simulink model "specificTaskTemplate"  (R2012b)
settings: Solver=FixedStepDiscrete  StartTime=0.0  StopTime=10.0  FixedStep=0.001  RelTol=1e-3
undefined symbols (not defined in the file): acquireMethods, clickPercentage, clickRefractoryPeriod, cuedText, cuedTextLength, cumulativeDwell, cursorDiameter, cursorDownColor, cursorNeuralColor, cursorNonneuralColor, displayShape, displayShape_1, displayShape_10, displayShape_2, displayShape_3, displayShape_4, displayShape_5, displayShape_6, displayShape_7, displayShape_8, displayShape_9, dwellRefractoryPeriod, gain, gloveBias, gloveLPDenominator, gloveLPNumerator, height, height_1, height_10, height_2, height_3, height_4, height_5, height_6, height_7, height_8, height_9, holdTime, ID, ID_1, ID_10, ID_2, ID_3, ID_4, ID_5, ID_6, ID_7, ID_8, ID_9, initialInput, initialLockout, initialState, inputType, keyboard, keyboardDims, keyPressedTime, maxTaskTime, mouseLPDenominator, mouseLPNumerator, mouseOffset ... (+122)
(part 2 of 2)

== matlab function specificTaskTemplate/keyboardTask ==
  data: xk input double size=[5 1]; behaviorPacket input Bus: behaviorPacketBus size=1; vizData input Bus: peripheralData; clickState input; clickParameters input; taskOutput output Bus: taskOutput; stateParameters input Bus: stateParams size=1; taskParameters input Bus: taskParamsBus; clock input; xpcTET input; keys input
function taskOutput  = keyboardTask(xk, behaviorPacket, vizData, clickState, clickParameters, stateParameters, taskParameters, clock, xpcTET, keys)
%#codegen

mouse = behaviorPacket.mouse(1:6);
glove = behaviorPacket.glove(1:5);
behaviorRequestClock = behaviorPacket.xpcRequestClock;
peripheralTimestamp = behaviorPacket.peripheralTimestamp(1:16);

%% CONSTANTS
TASK_NAME = 'keyboard';
VERSION_ID = single(2.010);
NUM_DIMS = double(DecoderConstants.NUM_KINEMATIC_DIMENSIONS);
STATEVEC_SIZE = 2*NUM_DIMS+1;
INIT_LENGTH = uint16(100); %ms
PRE_TRIAL_LENGTH = uint16(20); %ms
SCORE_LENGTH = uint16(4000); %ms
INIT_TIME = uint32(100);


%% INITIALIZE CURSOR TASK OUTPUT
fileLoggerData.data = uint8(zeros(1,1400));
fileLoggerData.dataLen = uint16(0);
fileLoggerData.fileName = uint8(zeros(1,20));
fileLoggerData.send = false;

fileLoggerFormat.format = uint8(zeros(1,1400));
fileLoggerFormat.formatLen = uint16(0);
fileLoggerFormat.fileName = uint8(zeros(1,20));

fileLoggerFormatAndData.format = fileLoggerFormat;
fileLoggerFormatAndData.data = fileLoggerData;

allowStop = true;
resetHMM = false;
taskOutput.flushFiles = false;
taskOutput.sendFormat = false;
taskOutput.taskDetails = fileLoggerFormat;
taskOutput.discrete = fileLoggerFormatAndData;
taskOutput.continuous = fileLoggerFormatAndData;
taskOutput.screen = fileLoggerFormatAndData;
taskOutput.sound = fileLoggerFormatAndData;
taskOutput.asynch = fileLoggerFormatAndData;
taskOutput.ttl = double(0);
taskOutput.xk = xk;
taskOutput.inputType = taskParameters.initialInput;
taskOutput.currentTarget = single(zeros([2 1]));
taskOutput.state = uint16(0);
taskOutput.paused = false;
taskOutput.allowStop = allowStop;
taskOutput.resetHMM = resetHMM;

%% TASK DETAILS PACKET
taskOutput.taskDetails = packFileLoggerTaskDetails(TASK_NAME, VERSION_ID, ...
    'STATE_INIT', uint8(KeyboardStates.STATE_INIT), ...
    'STATE_MOVE', uint8(KeyboardStates.STATE_MOVE),...
    'STATE_OVER_TARGET', uint8(KeyboardStates.STATE_OVER_TARGET),...
    'STATE_CLICK', uint8(KeyboardStates.STATE_CLICK),...
    'STATE_CLICK_REFRACTORY', uint8(KeyboardStates.STATE_CLICK_REFRACTORY),...
    'STATE_END', uint8(KeyboardStates.STATE_END),...
    'STATE_SHOW_SCORE', uint8(KeyboardStates.STATE_SHOW_SCORE),...
    'CLICK_IDLE', uint8(DiscreteStates.CLICK_IDLE),...
    'CLICK_MAIN', uint8(DiscreteStates.CLICK_MAIN),...
    'TASK_CUED_TEXT', uint8(keyboardConstants.TASK_CUED_TEXT), ...
    'TASK_FREE_TYPE', uint8(keyboardConstants.TASK_FREE_TYPE), ...
    'KEY_TYPE_LETTER', uint8(keyboardConstants.KEY_TYPE_LETTER), ...
    'KEY_TYPE_BACKSPACE', uint8(keyboardConstants.KEY_TYPE_BACKSPACE), ...
    'KEY_TYPE_SPACE', uint8(keyboardConstants.KEY_TYPE_SPACE), ...
    'KEY_TYPE_RETURN', uint8(keyboardConstants.KEY_TYPE_RETURN), ...
    'INPUT_TYPE_MOUSE_ABSOLUTE', uint8(cursorConstants.INPUT_TYPE_MOUSE_ABSOLUTE), ...
    'INPUT_TYPE_DECODE_V', uint8(cursorConstants.INPUT_TYPE_DECODE_V),...
    'CLICK_TYPE_NONE', uint8(clickConstants.CLICK_TYPE_NONE),...
    'CLICK_TYPE_GLOVE', uint8(clickConstants.CLICK_TYPE_GLOVE),...
    'CLICK_TYPE_NEURAL', uint8(clickConstants.CLICK_TYPE_NEURAL)...
);



%% DEFINE PERSISTENTS
persistent state vizPacket;
persistent pauseTriggered;
persistent stateTimer;
persistent holdTimer;
persistent cursorColor;

persistent trialNum;
persistent textInd;

persistent lockedParameters inputType;

persistent textSequence;
persistent previousOverTarget;
persistent selectedTarget;

persistent lastSoundTime lastSoundState lastAcquireMethod;

persistent totalTaskTime;

persistent lastResetTime lastResetState;
persistent initialClickTimer;

persistent lastEnteredCharacter;

%% store the amount of time dwelled on any target
persistent cumulativeDwell;

persistent lastRecenterTime lastRecenterSpot;

%% INITIALIZE PERSISTENTS
if(isempty(state))
    state = uint16(KeyboardStates.STATE_INIT);
    
    vizPacket = initVizPacket;
    stateTimer = uint16(0);
    holdTimer = uint16(0);
    pauseTriggered = true;
    
    cursorColor = double(zeros([3 1]));
    
    xk = double(zeros([STATEVEC_SIZE 1]));
    xk(end,1) = 1;
    
    %% buffer all the parameters off the bus
    lockedParameters = taskParameters;
    inputType = lockedParameters.initialInput;
    
    trialNum = uint16(1);
    textInd = uint16(1);
    previousOverTarget = uint16(0);
    selectedTarget = uint16(0);
    
    textSequence = zeros([1 uint16(keyboardConstants.MAX_CUED_TEXT)],'uint8');

    lastSoundTime = clock;
    lastSoundState = uint8(KeyboardStates.SOUND_STATE_IDLE);
    lastAcquireMethod = uint8(0);
    
    totalTaskTime = uint32(0);
    lastResetState = false;
    lastResetTime = uint32(0);
    initialClickTimer = uint16(0);
    lastEnteredCharacter = uint8(0);
    
	cumulativeDwell = initCumulativeDwell();
    lastRecenterTime = clock;
    lastRecenterSpot = [0;0];
end

%% trigger display resets on the rising edge of the parameter setting
resetDisplay = lockedParameters.resetDisplay;
if resetDisplay && ~lastResetState
    lastResetTime = clock;
end
lastResetState = resetDisplay;

if(clock < INIT_TIME)
    pauseTriggered = true;
end

if ~pauseTriggered
    totalTaskTime = totalTaskTime+1;
end
% We usually shouldn't write discrete data
writeDiscreteData = false;
writeContinuousData = true;

if(vizData.receive && (vizData.dataLen > 0 ))
    vizPacket = parseVizPacket(vizData.data);
end

isNeural = (uint16(inputType) == uint16(cursorConstants.INPUT_TYPE_DECODE_V));
isClicked = (uint16(clickState) == uint16(DiscreteStates.CLICK_MAIN));
isNone = (uint16(inputType) == uint16(cursorConstants.INPUT_TYPE_NONE));

%% set the cursor color 
%if isClicked
%    cursorColor(1:end) = taskParameters.cursorDownColor;
%else
if isNeural
    cursorColor(1:end) = taskParameters.cursorNeuralColor;
elseif isNone
    cursorColor(1:end) = [0; 204; 102;];
else
    cursorColor(1:end) = taskParameters.cursorNonneuralColor;
end

overTarget = uint16(0);
cuedTarget = uint16(0);
overCuedTarget = uint16(0);
cuedSuccess = uint8(0);
xkshift = xk(1:2)+[lockedParameters.xyOffset(1); lockedParameters.xyOffset(2)];

startStopTargetInd = uint8(keyboardConstants.KEY_INDEX_STARTSTOP);
startStopTarget = findKeyByLetter(keys,startStopTargetInd);

%% STATE MACHINE
switch state
    case {KeyboardStates.STATE_INIT}
        %% set all the persistents that may have been changed by user input
        pauseTriggered = stateParameters.pause;
        if ~mod(clock,300)
            lockedParameters = taskParameters;
        end
        %% do this every 300 ms to try to avoid partial parameter updates
        inputType = lockedParameters.initialInput;
        %% generate some entropy
        jnk = rand(1,1);
        
        stateTimer = stateTimer + 1;
        if stateTimer >= INIT_LENGTH
            xkshift = [0;0] + [lockedParameters.xyOffset(1); lockedParameters.xyOffset(2)] + double(lockedParameters.recenterOffset(:));
            if ~pauseTriggered
                inputType = lockedParameters.inputType;
                stateTimer = uint16(0);
                trialNum = uint16(1);
                state = uint16(lockedParameters.initialState);%uint16(KeyboardStates.STATE_MOVE);
                writeDiscreteData = true;
                lockedParameters = taskParameters;
           end
        end
    case {KeyboardStates.STATE_INACTIVE}
        stateTimer = stateTimer + 1;
        if stateTimer > lockedParameters.dwellRefractoryPeriod
            cuedTarget = startStopTarget;
            overTarget = isCursorOverTarget(keys, xkshift, lockedParameters.keyboardDims,...
                lockedParameters.showBackspace, lockedParameters.showStartStop);
            
            %% if over the target
            if overTarget == cuedTarget
                holdTimer = holdTimer+uint16(1);
                if clickState == uint16(DiscreteStates.CLICK_MAIN)
                    initialClickTimer = initialClickTimer + uint16(1);
                end
            else
                holdTimer=uint16(0);
                initialClickTimer = uint16(0);
            end
            
            targetAcquired = false;
            %% check the acquire methods
            if (bitand(lockedParameters.acquireMethods, uint8(keyboardConstants.ACQUIRE_DWELL)) ...
                    && holdTimer > lockedParameters.holdTime)
                targetAcquired = true;
                lastAcquireMethod = uint8(keyboardConstants.ACQUIRE_DWELL);
            elseif(bitand(lockedParameters.acquireMethods, uint8(keyboardConstants.ACQUIRE_CLICK)) ...
                    && initialClickTimer > clickParameters.clickHoldTime)
                targetAcquired = true;
                lastAcquireMethod = uint8(keyboardConstants.ACQUIRE_CLICK);
            end
            
            if targetAcquired
                selectedTarget = overTarget;
                state = uint16(KeyboardStates.STATE_DWELL_REFRACTORY);
                stateTimer = uint16(0);
                holdTimer = uint16(0);
                cumulativeDwell = initCumulativeDwell();
                initialClickTimer = uint16(0);
                trialNum = trialNum + 1;
                writeDiscreteData = true;
                lockedParameters = taskParameters;
                lastSoundTime = clock;
                lastSoundState = uint8(KeyboardStates.SOUND_STATE_CLICK);
            end
        end
    case {KeyboardStates.STATE_MOVE}
        stateTimer = stateTimer + 1;
        
        if lockedParameters.taskType == uint8(keyboardConstants.TASK_CUED_TEXT)
            cuedLetter = uint8(lockedParameters.cuedText(textInd));
            cuedTarget = findKeyByLetter(keys,cuedLetter);
        end
        overTarget = isCursorOverTarget(keys, xkshift, lockedParameters.keyboardDims,...
            lockedParameters.showBackspace, lockedParameters.showStartStop);
        
        if overTarget == cuedTarget
            overCuedTarget = overTarget;
        end
        if overTarget && totalTaskTime > lockedParameters.initialLockout
            state = uint16(KeyboardStates.STATE_OVER_TARGET);
            holdTimer = uint16(0);
            lastSoundTime = clock;
            lastSoundState = uint8(KeyboardStates.SOUND_STATE_OVER_TARGET);
        elseif stateTimer >= lockedParameters.trialTimeout
            %% timeout - go to the next target
            if cuedTarget && lockedParameters.recenterOnFail
                if lockedParameters.recenterFullscreen
                    xkshift = [0;0] + [lockedParameters.xyOffset(1); lockedParameters.xyOffset(2)] + double(lockedParameters.recenterOffset(:));
                else
                    xkshift(1) = double(keys.x(cuedTarget)) + double(keys.width(cuedTarget))/2;
                    xkshift(2) = double(keys.y(cuedTarget)) + double(keys.height(cuedTarget))/2;
                end
                lastRecenterTime = clock;
                lastRecenterSpot = xkshift;
            end
            stateTimer = uint16(0);
            holdTimer = uint16(0);
            cumulativeDwell = initCumulativeDwell();
            state = uint16(KeyboardStates.STATE_MOVE);
            trialNum = trialNum + 1;
            writeDiscreteData = true;
            lockedParameters = taskParameters;
        end
        %% refractory states to prevent repeated clicks...
    case {KeyboardStates.STATE_KEY_PRESSED}
        stateTimer = stateTimer+1;
                
        %% highlight cued target if needed
        if lockedParameters.taskType == uint8(keyboardConstants.TASK_CUED_TEXT)
            cuedLetter = char(lockedParameters.cuedText(textInd));
            cuedTarget = findKeyByLetter(keys,cuedLetter);
        end
        if stateTimer > lockedParameters.keyPressedTime
            selectedTarget = uint16(0);
            if lastAcquireMethod == uint8(keyboardConstants.ACQUIRE_DWELL)
                %% in case of dwell
                if stateTimer < lockedParameters.dwellRefractoryPeriod
                    state = uint16(KeyboardStates.STATE_DWELL_REFRACTORY);
                else
                    stateTimer = uint16(0);
                    state = uint16(KeyboardStates.STATE_MOVE);
                end
            else
                %% in case of click
                if stateTimer < lockedParameters.clickRefractoryPeriod
                    state = uint16(KeyboardStates.STATE_CLICK_REFRACTORY);
                else
                    stateTimer = uint16(0);
                    state = uint16(KeyboardStates.STATE_MOVE);
                end
            end
        end
        
        %% refractory states to prevent repeated clicks...
    case {KeyboardStates.STATE_CLICK_REFRACTORY}
        stateTimer = stateTimer+1;
        % no need to allow cursor stoppage during click refrac
        allowStop = false;
        % ensure click state is false during refractory period
        resetHMM = true;
        if lockedParameters.taskType == uint8(keyboardConstants.TASK_CUED_TEXT)
            cuedLetter = char(lockedParameters.cuedText(textInd));
            cuedTarget = findKeyByLetter(keys,cuedLetter);
        end
        if stateTimer > lockedParameters.clickRefractoryPeriod
            stateTimer = uint16(0);
            state = uint16(KeyboardStates.STATE_MOVE);
        end            
    case {KeyboardStates.STATE_DWELL_REFRACTORY}
        stateTimer = stateTimer+1;
        % no need to allow cursor stoppage during dwell refrac
        allowStop = false;
        % ensure click state is false during refractory period
        resetHMM = true;
        if lockedParameters.taskType == uint8(keyboardConstants.TASK_CUED_TEXT)
            cuedLetter = char(lockedParameters.cuedText(textInd));
            cuedTarget = findKeyByLetter(keys,cuedLetter);
        end
        if stateTimer > lockedParameters.dwellRefractoryPeriod
            stateTimer = uint16(0);
            state = uint16(KeyboardStates.STATE_MOVE);
        end            
        
    case {KeyboardStates.STATE_OVER_TARGET}
        stateTimer = stateTimer + 1;
        holdTimer = holdTimer + 1;
        if lockedParameters.taskType == uint8(keyboardConstants.TASK_CUED_TEXT)
            cuedLetter = char(lockedParameters.cuedText(textInd));
            cuedTarget = findKeyByLetter(keys,cuedLetter);
        end
        overTarget = isCursorOverTarget(keys, xkshift, lockedParameters.keyboardDims, lockedParameters.showBackspace, lockedParameters.showStartStop);
        % increment the cumulative dwell counter for this target
        if overTarget, cumulativeDwell(overTarget) = cumulativeDwell(overTarget)+1; end
        if overTarget == cuedTarget
            overCuedTarget = overTarget;
        end
        if ~overTarget
            % not over any target. reset stuff on the way out of this state.
            state = uint16(KeyboardStates.STATE_MOVE);
            holdTimer = uint16(0);
            stateTimer = uint16(0);
        elseif overTarget ~= previousOverTarget
            holdTimer = uint16(0);
            lastSoundTime = clock;
            lastSoundState = uint8(KeyboardStates.SOUND_STATE_OVER_TARGET);
        elseif (bitand(lockedParameters.acquireMethods, uint8(keyboardConstants.ACQUIRE_DWELL)) ...
                && (holdTimer > lockedParameters.holdTime || (lockedParameters.cumulativeDwell && cumulativeDwell(overTarget) >= lockedParameters.holdTime))) 
            %% acquired some kinda target.
            if overTarget == startStopTarget;
                % special case - stop the keyboard
                state = uint16(KeyboardStates.STATE_INACTIVE);
                stateTimer = uint16(0);
                holdTimer = uint16(0);
                cumulativeDwell = initCumulativeDwell();
                trialNum = trialNum + 1;
                writeDiscreteData = true;
                lockedParameters = taskParameters;
                lastSoundTime = clock;
                lastAcquireMethod = uint8(keyboardConstants.ACQUIRE_DWELL);
                lastSoundState = uint8(KeyboardStates.SOUND_STATE_CLICK);
            else
                %% OK, process the selection.
                [textSequence, textInd] = applyLetter(textSequence, textInd, keys, ...
                    overTarget);
                if textInd >2
                    if keys.type(overTarget) == keyboardConstants.KEY_TYPE_SPACE
                        if lastEnteredCharacter == uint8(' ')
                            textSequence(textInd-2) = '.';
                        end
                    end
                end
                lastEnteredCharacter = textSequence(textInd-1);
                
                if overCuedTarget
                    cuedSuccess = uint8(1);
                end
                if ~cuedSuccess && lockedParameters.recenterOnFail || ...
                        cuedSuccess && lockedParameters.recenterOnSuccess
                    if lockedParameters.recenterFullscreen
                        xkshift = [0;0] + [lockedParameters.xyOffset(1); lockedParameters.xyOffset(2)] + double(lockedParameters.recenterOffset(:));
                    else
                        xkshift(1) = double(keys.x(cuedTarget)) + double(keys.width(cuedTarget))/2;
                        xkshift(2) = double(keys.y(cuedTarget)) + double(keys.height(cuedTarget))/2;
                    end
                    lastRecenterTime = clock;
                    lastRecenterSpot = xkshift;
               end
                selectedTarget = overTarget;
                %  state = uint16(KeyboardStates.STATE_DWELL_REFRACTORY);
                state = uint16(KeyboardStates.STATE_KEY_PRESSED);
                stateTimer = uint16(0);
                holdTimer = uint16(0);
                cumulativeDwell = initCumulativeDwell();
                trialNum = trialNum + 1;
                writeDiscreteData = true;
                lockedParameters = taskParameters;
                lastSoundTime = clock;
                lastAcquireMethod = uint8(keyboardConstants.ACQUIRE_DWELL);
                if ~cuedSuccess && lockedParameters.soundOnError
                    lastSoundState = uint8(KeyboardStates.SOUND_STATE_ERROR);
                else
                    lastSoundState = uint8(KeyboardStates.SOUND_STATE_CLICK);
                end
            end
        elseif (bitand(lockedParameters.acquireMethods, uint8(keyboardConstants.ACQUIRE_CLICK)) ...
                && clickState == uint16(DiscreteStates.CLICK_MAIN))
            %% we were resetting holdTimer to 1 at this stage but that seems silly. - CP 20141118
            % holdTimer = uint16(1); 
            stateTimer = uint16(0);
            state = uint16(KeyboardStates.STATE_CLICK);            
        end
    case {KeyboardStates.STATE_CLICK}
        stateTimer = stateTimer + 1;
        holdTimer = holdTimer + 1;
        if lockedParameters.taskType == uint8(keyboardConstants.TASK_CUED_TEXT)
            cuedLetter = char(lockedParameters.cuedText(textInd));
            cuedTarget = findKeyByLetter(keys,cuedLetter);
        end
        overTarget = isCursorOverTarget(keys, xkshift, lockedParameters.keyboardDims, lockedParameters.showBackspace, lockedParameters.showStartStop);
        if overTarget, cumulativeDwell(overTarget) = cumulativeDwell(overTarget)+1; end
        if overTarget == cuedTarget
            overCuedTarget = overTarget;
        end
        if ~overTarget
            % no longer over a target. reset stuff on the way out.
            state = uint16(KeyboardStates.STATE_MOVE);
            holdTimer = uint16(0);
            stateTimer = uint16(0);
        elseif overTarget ~= previousOverTarget
            % over a new target. reset stuff.
            holdTimer = uint16(0);
            stateTimer = uint16(0);
        end
        if clickState ~= uint16(DiscreteStates.CLICK_MAIN)
            % no longer clicking, so we must be leaving this state
            stateTimer = uint16(0);
            if overTarget
                state = uint16(KeyboardStates.STATE_OVER_TARGET);
            else
                holdTimer = uint16(0);
                state = uint16(KeyboardStates.STATE_MOVE);
            end
        end
        %% this timing used to be done with 'holdTimer', now that is stateTimer - CP 20141118
        % if overTarget && holdTimer >= clickParameters.clickHoldTime 
        if overTarget && stateTimer >= clickParameters.clickHoldTime 
            if overTarget == startStopTarget;
                % special case : stop the keyboard
                state = uint16(KeyboardStates.STATE_INACTIVE);
                stateTimer = uint16(0);
                holdTimer = uint16(0);
                cumulativeDwell = initCumulativeDwell();
                trialNum = trialNum + 1;
                writeDiscreteData = true;
                lockedParameters = taskParameters;
                lastSoundTime = clock;
                lastAcquireMethod = uint8(keyboardConstants.ACQUIRE_DWELL);
                lastSoundState = uint8(KeyboardStates.SOUND_STATE_CLICK);
            else
                %% acquired some kinda target.
                [textSequence, textInd] = applyLetter(textSequence, textInd, keys, ...
                    overTarget);
                if textInd >2
                    if keys.type(overTarget) == keyboardConstants.KEY_TYPE_SPACE
                        if lastEnteredCharacter == uint8(' ')
                            textSequence(textInd-2) = '.';
                        end
                    end
                end
                lastEnteredCharacter = textSequence(textInd-1);
                if overCuedTarget
                    cuedSuccess = uint8(1);
                end
                if ~cuedSuccess && lockedParameters.recenterOnFail || ...
                        cuedSuccess && lockedParameters.recenterOnSuccess
                    if lockedParameters.recenterFullscreen
                        xkshift = [0;0] + [lockedParameters.xyOffset(1); lockedParameters.xyOffset(2)] + double(lockedParameters.recenterOffset(:));
                    else
                        xkshift(1) = double(keys.x(cuedTarget)) + double(keys.width(cuedTarget))/2;
                        xkshift(2) = double(keys.y(cuedTarget)) + double(keys.height(cuedTarget))/2;
                    end
                    lastRecenterTime = clock;
                    lastRecenterSpot = xkshift;
                end
                % state = uint16(KeyboardStates.STATE_CLICK_REFRACTORY);
                selectedTarget = overTarget;
                state = uint16(KeyboardStates.STATE_KEY_PRESSED);
                stateTimer = uint16(0);
                holdTimer = uint16(0);
                cumulativeDwell = initCumulativeDwell();
                trialNum = trialNum+1;
                writeDiscreteData = true;
                lockedParameters = taskParameters;
                lastSoundTime = clock;
                lastAcquireMethod = uint8(keyboardConstants.ACQUIRE_CLICK);
                %% if there is an error and we want error sounds, make error sound.
                if ~cuedSuccess && lockedParameters.soundOnError
                    lastSoundState = uint8(KeyboardStates.SOUND_STATE_ERROR);
                else
                    lastSoundState = uint8(KeyboardStates.SOUND_STATE_CLICK);
                end
            end
        elseif stateTimer >= lockedParameters.trialTimeout
            %% timeout - go to the next target
            if cuedTarget && lockedParameters.recenterOnFail
                if lockedParameters.recenterFullscreen
                    xkshift = [0;0] + [lockedParameters.xyOffset(1); lockedParameters.xyOffset(2)] + double(lockedParameters.recenterOffset(:));
                else
                    xkshift(1) = double(keys.x(cuedTarget)) + double(keys.width(cuedTarget))/2;
                    xkshift(2) = double(keys.y(cuedTarget)) + double(keys.height(cuedTarget))/2;
                end
                lastRecenterTime = clock;
                lastRecenterSpot = xkshift;
            end
            stateTimer = uint16(0);
            holdTimer = uint16(0);
            cumulativeDwell = initCumulativeDwell();
            state = uint16(KeyboardStates.STATE_MOVE);
            trialNum = trialNum + 1;
            writeDiscreteData = true;
            lockedParameters = taskParameters;
        end
        
    case {KeyboardStates.STATE_SHOW_SCORE}
        stateTimer = stateTimer + 1;
        if stateTimer >= lockedParameters.scoreTime
            state = uint16(KeyboardStates.STATE_END);
            stateTimer = uint16(0);
        end
        
    case {KeyboardStates.STATE_END}
        stateTimer = stateTimer + 1;
        
end

if lockedParameters.maxTaskTime && totalTaskTime > lockedParameters.maxTaskTime
    state = uint16(KeyboardStates.STATE_END);
end

%% lock cursor if desired
if (lockedParameters.recenterDelay>0) && ...
        (clock - lastRecenterTime < lockedParameters.recenterDelay)
    xkshift = lastRecenterSpot;
end



previousOverTarget = overTarget;
taskOutput.xk(1:2) = xkshift -[lockedParameters.xyOffset(1); lockedParameters.xyOffset(2)];
taskOutput.state = state;
if cuedTarget
    taskOutput.currentTarget(1) = double(keys.x(cuedTarget)) + double(keys.width(cuedTarget))/2;
    taskOutput.currentTarget(2) = double(keys.y(cuedTarget)) + double(keys.height(cuedTarget))/2;
end

%% PACK DATA FOR UDP OUTPUT
taskOutput.continuous = packFileLoggerFormatAndData('continuous', ...
    TASK_NAME, VERSION_ID, ...
    'clock', clock, ...
    'pause', pauseTriggered, ...
    'xpcRequestClock', behaviorRequestClock, ...
    'peripheralTimestamp', peripheralTimestamp, ...
    'state', state, ...
    'inputType', inputType, ...
    'mouse', mouse, ...
    'glove', glove, ...
    'gloveRL', behaviorPacket.gloveSerial(6), ...
    'glove2', behaviorPacket.glove2, ...
    'gloveRL2', behaviorPacket.gloveSerial2(6), ...
    'peripheralTimestamp', peripheralTimestamp,...
    'xpcScreenUpdateClock',vizPacket.xpcScreenUpdateClock,...
    'cursorPosition', single(xkshift(1:2)), ...
    'cuedTarget', cuedTarget,...
    'overTarget', overTarget,...
    'overCuedTarget', overCuedTarget,...
    'clickState', uint16(clickState),...
    'xk', single(taskOutput.xk),...
    'stateTimer', stateTimer, ...
    'holdTimer', holdTimer, ...
    'xpcTET', single(xpcTET) ...
    );




%% SEND DISCRETE DATA TO FILELOGGER
taskOutput.discrete = packFileLoggerFormatAndData('discrete', ...
    TASK_NAME, VERSION_ID, ...
    'clock', clock,...
    'blockNumber', stateParameters.blockNumber,...
    'state', state, ...
    'cuedSuccess',cuedSuccess,...
    'keyboard',lockedParameters.keyboard,...
    'keyboardDims',lockedParameters.keyboardDims,...
    'cuedTarget', cuedTarget,...
    'clickSource',clickParameters.clickSource,...
    'clickHoldTime',clickParameters.clickHoldTime,...
    'hmmClickLikelihoodThreshold',clickParameters.hmmClickLikelihoodThreshold,...
    'gloveThreshold',clickParameters.gloveThreshold,...
    'gloveIndices',clickParameters.gloveIndices,...
    'gloveBias',lockedParameters.gloveBias,...
    'cursorDiameter', lockedParameters.cursorDiameter,...
    'workspaceX', lockedParameters.workspaceX,...
    'workspaceY', lockedParameters.workspaceY,...
    'xyOffset', lockedParameters.xyOffset,...
    'recenterOnSuccess', lockedParameters.recenterOnSuccess,...
    'recenterOnFail', lockedParameters.recenterOnFail,...
    'recenterDelay', lockedParameters.recenterDelay,...
    'clickRefractoryPeriod', lockedParameters.clickRefractoryPeriod,...
    'dwellRefractoryPeriod', lockedParameters.dwellRefractoryPeriod,...
    'useGloveLPF', uint8(lockedParameters.useGloveLPF),...
    'hmmClickSpeedMax',single(clickParameters.hmmClickSpeedMax),...
    'stopOnClick', lockedParameters.stopOnClick,...
    'showBackspace',lockedParameters.showBackspace,...
    'showTargetText',lockedParameters.showTargetText,...
    'showTypedText',lockedParameters.showTypedText,...
    'showCueOnTarget',lockedParameters.showCueOnTarget,...
    'cumulativeDwell',lockedParameters.cumulativeDwell,...
    'key1params',single([keys.x(1) keys.y(1) keys.width(1) keys.height(1)]),...
    'taskType', lockedParameters.taskType ...
   );
%    'gloveLPNumerator', single(lockedParameters.gloveLPNumerator), ...
%    'gloveLPDenominator', single(lockedParameters.gloveLPNumerator), ...


%% SEND DATA OUT TO VIZ
taskOutput.screen = packFileLoggerFormatAndData('screen', ...
    TASK_NAME, VERSION_ID, ...
    'clock', clock,...
    'totalTaskTime',totalTaskTime,...
    'blockNumber', stateParameters.blockNumber,...
    'state',state,...
    'keyboard',lockedParameters.keyboard,...
    'keyboardDims',lockedParameters.keyboardDims,...
    'showBackspace',lockedParameters.showBackspace,...
    'showStartStop',lockedParameters.showStartStop,...
    'cursorPosition', xkshift(1:2),...
    'cursorColor', cursorColor,...
    'cuedTarget', cuedTarget,...
    'overTarget', overTarget,...
    'overCuedTarget', overCuedTarget,...
    'selectedTarget', selectedTarget,...
    'textInd',textInd,...
    'trialNum',trialNum,...
    'lastAcquireMethod',lastAcquireMethod,...
    'resetDisplay',resetDisplay,...
    'lastResetTime',lastResetTime,...
    'showStartStop',lockedParameters.showStartStop,...
    'numKeys',keys.numKeys(1),...
    'cursorDiameter', lockedParameters.cursorDiameter,...
    'inputType', inputType,...
    'cuedText',uint8(lockedParameters.cuedText(1:140)),...
    'cuedTextLength',uint8(lockedParameters.cuedTextLength),...
    'textSequence', textSequence,...
    'showTargetText',lockedParameters.showTargetText,...
    'showTypedText',lockedParameters.showTypedText,...
    'showCueOnTarget',lockedParameters.showCueOnTarget,...
    'showCueOffTarget',lockedParameters.showCueOffTarget,...
    'lastAcquireMethod',lastAcquireMethod,...
    'taskType', lockedParameters.taskType...
    );


%% SEND DATA OUT TO SOUND
taskOutput.sound = packFileLoggerFormatAndData('screen', ...
    TASK_NAME, VERSION_ID, ...
    'clock', clock,...
    'vizState',state,...
    'acquireMethod',lastAcquireMethod,...
    'lastSoundTime',lastSoundTime,...
    'lastSoundState',lastSoundState...
    ); 


%% SET SEND FLAGS FOR NETWORK OUTPUTS
if(clock < INIT_TIME)
    taskOutput.discrete.data.send = false;
    taskOutput.continuous.data.send = false;
    taskOutput.screen.data.send = false;
    taskOutput.sound.data.send = false;
    
    if(mod(clock, 10)==0)
        taskOutput.sendFormat = true;
    else
        taskOutput.sendFormat = false;
    end
    stateTimer = uint16(0);
else
    taskOutput.discrete.data.send = writeDiscreteData;
    taskOutput.continuous.data.send = writeContinuousData;
    taskOutput.screen.data.send = true;
    taskOutput.sound.data.send = true;
    taskOutput.sendFormat = false;
    taskOutput.inputType = inputType;
end

taskOutput.allowStop = allowStop;
taskOutput.resetHMM = resetHMM;
taskOutput.paused = pauseTriggered;

end



function vizPacket = parseVizPacket(packetData)

    vizPacket.xpcScreenUpdateClock = typecast(packetData(28+[1:4]), 'uint32');

end

function vizPacket = initVizPacket()

    vizPacket.xpcScreenUpdateClock = uint32(0);

end

function [textIn, newInd] = applyLetter(textIn, currentInd, keys, whichKey)
    newInd = currentInd;
    switch keys.type(whichKey)
      case {keyboardConstants.KEY_TYPE_LETTER, keyboardConstants.KEY_TYPE_SPACE}
        textIn(currentInd) = keys.text(whichKey);
        newInd = currentInd+1;
      case {keyboardConstants.KEY_TYPE_BACKSPACE}
          if currentInd>1
            textIn(currentInd-1) = 0;
            newInd = currentInd-1;
          end
    end
end


function x = initCumulativeDwell()
    x = zeros([1 uint16(keyboardConstants.MAX_NUM_KEYS)],'uint16');
end
